simulink model "entryVehicle"  (R2025a)
settings: Solver=ode5  StartTime=startTime  StopTime=stopTime  FixedStep=stepTime  RelTol=1e-3
values from neighbouring files (symbols this model uses):
  alpha_0 = deg2rad(-23.)    [run_entryVehicle.m]
  alpha_T_CD = [0 5 10 15 20 25 30 35 40]    [ApolloDragCoeff.mat]
  alpha_T_CL = [0 5 10 15 20 25 30 35 40]    [ApolloLiftCoeff.mat]
  beta_0 = deg2rad(0.05)    [run_entryVehicle.m]
  CD_T = [1.13 1.305 1.34 1.394 1.445 1.472 1.48 1.468 1.454 1.486 1.51 1.124 ... (99 elements, 11x9)]    [ApolloDragCoeff.mat]
  chi_0 = deg2rad(90)    [run_entryVehicle.m]
  CL_T = [0 0 0 0 0 0 0 0 0 0 0 0.098 ... (99 elements, 11x9)]    [ApolloLiftCoeff.mat]
  d_ref = 3.9    [run_entryVehicle.m]
  gamma_0 = deg2rad(-9.536)    [run_entryVehicle.m]
  H_s = 7050    [run_entryVehicle.m]
  I_xx = 5617.61    [run_entryVehicle.m]
  I_xz = 0    [run_entryVehicle.m]
  I_yy = 4454.62    [run_entryVehicle.m]
  I_zz = 4454.80    (= 4454.8)    [run_entryVehicle.m]
  lambda_0 = deg2rad(0)    [run_entryVehicle.m]
  m_0 = 4976    [run_entryVehicle.m]
  Mach_numbers_CD = [0.9 1.1 1.2 1.35 1.65 2 2.4 3 4 6 10]    [ApolloDragCoeff.mat]
  Mach_numbers_CL = [0.9 1.1 1.2 1.35 1.65 2 2.4 3 4 6 10]    [ApolloLiftCoeff.mat]
  Mars_mu = 3.98319648e14    (= 398319648000000)    [run_entryVehicle.m]
  Mars_radius = 6371e3    (= 6371000)    [run_entryVehicle.m]
  p_0 = deg2rad(0)    [run_entryVehicle.m]
  q_0 = deg2rad(0)    [run_entryVehicle.m]
  r_0 = deg2rad(0)    [run_entryVehicle.m]
  R_0 = 220e3 + Mars_radius    (= 6591000)    [run_entryVehicle.m]
  r_cm = [1.57; 0; -0.137]    [run_entryVehicle.m]
  R_s = 287    [run_entryVehicle.m]
  rho_0 = 1.225    [run_entryVehicle.m]
  S_ref = 12    [run_entryVehicle.m]
  sigma_0 = deg2rad(110.)    [run_entryVehicle.m]
  specific_heat = 1.33    [run_entryVehicle.m]
  stepTime = 0.01    [run_entryVehicle.m]
  tau_0 = deg2rad(0)    [run_entryVehicle.m]
  V_0 = 11e3    (= 11000)    [run_entryVehicle.m]
undefined symbols (not defined in the file or in its folder): A_attitude, acce_bias, acce_S, alpha_T_Cm, alpha_T_Cm_q, B_attitude, Cm_qT, Cm_T, dynamics_constants, K_lat, K_long, lateral_ref, longitudinal_ref, Mach_numbers_Cm, Mach_numbers_Cm_q, my_max, Q0, r0_eci, rateGyro_bias, rateGyro_S, v0_eci
libraries: simulink_extras x32, simulink x3, SignalEditorBlockLib x1
(part 3 of 3)

== matlab function entryVehicle/Plant/Kinematics/Translation Kinematics/MATLAB Function ==
  data: R_dot output; tau_dot output; lambda_dot output; V input; gamma input; chi input; R input; lambda input
function [R_dot, tau_dot, lambda_dot] = Translation_Kinematics(V, gamma, chi, R, lambda)

R_dot = V * sin(gamma);
tau_dot = (V * cos(gamma) * sin(chi)) / (R * cos(lambda));
lambda_dot = V / R * cos(gamma) * cos(chi);

== matlab function entryVehicle/Plant/Kinematics/Attitude Kinematics/MATLAB Function1 ==
  data: L input; S input; p input; q input; alpha_dot output; beta_dot output; sigma_dot output; r input; alpha input; beta input; sigma input; m input; g input; V input; gamma input
function [alpha_dot, beta_dot, sigma_dot] = Attitude_Kinematics(L, S, p, q, r, alpha, beta, sigma, m, g, V, gamma)

alpha_dot = q - (p*cos(alpha) + r*sin(alpha))*tan(beta) - (L - m*g*cos(gamma)*cos(sigma))/(m*V*cos(beta));
%alpha_dot = q - (p*cos(alpha) + r*sin(alpha))*tan(beta);
beta_dot = p*sin(alpha) - r*cos(alpha) - (S + m*g*cos(gamma)*sin(sigma))/(m*V);
%beta_dot = p*sin(alpha) - r*cos(alpha);
sigma_dot = -(p*cos(alpha) + r*sin(alpha))/(cos(beta)) - (L - m*g*cos(gamma)*cos(sigma))/(m*V)*tan(beta) + (L*sin(sigma) + S*cos(sigma))/(m*V)*tan(gamma);
%sigma_dot = -(p*cos(alpha) + r*sin(alpha))/(cos(beta));

if ~isfinite(alpha_dot)
    disp('Non-finite alpha_dot at t=0');
end

if any(~isfinite([L, S, p, q, r, alpha, beta, sigma, m, g, V, gamma]))
    disp('Invalid input at t=0:');
    disp([L, S, p, q, r, alpha, beta, sigma, m, g, V, gamma]);
end
